simulink model "lqr_period_with_r_and_d_simulink"  (R2015a)
settings: Solver=ode45  SolverMode=SingleTasking  StartTime=0.0  StopTime=simu.time  RelTol=1e-3
values from neighbouring files (symbols this model uses):
  plant = tf([10],[tau 1])    [lqr_period_with_abitary_reference.m]
undefined symbols (not defined in the file or in its folder): simu
undefined symbols (not defined in the file): parameters
libraries: simulink x1
settings Model: CovSFcnEnable=off  ExtModeTrigMode=oneshot  ExtModeArmWhenConnect=off  Creator=The MathWorks Inc.  LastModifiedBy=Xiaotian
settings DataIOCC: LimitDataPoints=off  SaveOutput=off  SignalLogging=off  DSMLogging=off  SaveTime=off  SignalLoggingName=sigsOut
settings OptimizationCC: BooleanDataType=off  ExpressionDepthLimit=2147483647  InitFltsAndDblsToZero=on
settings DebuggingCC: SaveWithParameterizedLinksMsg=none  UnderspecifiedInitializationDetection=Classic  MergeDetectMultiDrivingBlocksExec=none  SignalResolutionControl=TryResolveAllWithWarning  MultiTaskDSMMsg=warning  MultiTaskCondExecSysMsg=none  IntegerOverflowMsg=none  FcnCallInpInsideContextMsg=UseLocalSettings  StateNameClashWarn=warning  IntegerSaturationMsg=none
settings HardwareCC: TargetUnknown=on
settings GRTTargetCC: TargetFcnLib=ansi_tfl_tmw.mat  CombineOutputUpdateFcns=off  GRTInterface=on

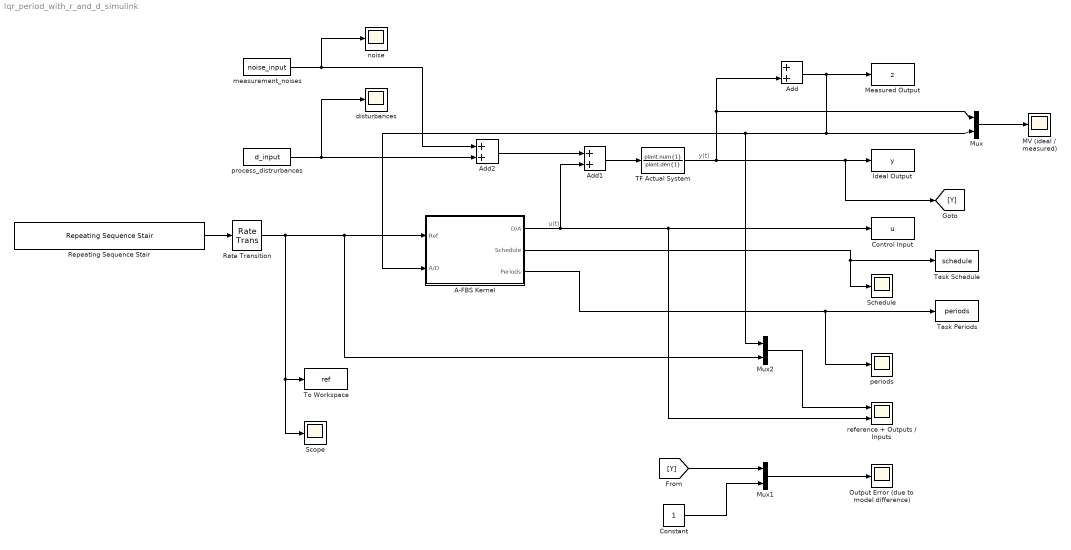
== system lqr_period_with_r_and_d_simulink ==
  note: u(t)
  note: y(t)
  A-FBS Kernel : Subsystem  mask{afbs_para=parameters}
      mask prompts: afbs_para "A-FBS Parameters"
  Add : Sum
  Add1 : Sum
  Add2 : Sum
  Constant : Constant
  Control Input : ToWorkspace  VariableName=u  SampleTime=simu.samlping_time
      settings: MaxDataPoints=Inf
  Ideal Output : ToWorkspace  VariableName=y  SampleTime=simu.samlping_time
      settings: MaxDataPoints=Inf
  MV (ideal / measured) : Scope
      settings: TimeRange=10  YMin=-1.5  YMax=1.75  DataFormat=Structure
  Measured Output : ToWorkspace  VariableName=z  SampleTime=simu.samlping_time
      settings: MaxDataPoints=Inf
  Mux : Mux  Inputs=2
  Mux1 : Mux  Inputs=2
  Mux2 : Mux  Inputs=2
  Output Error (due to model difference) : Scope
      settings: TimeRange=10  YMin=-29.95  YMax=-29.6  SaveName=ScopeData2  DataFormat=Structure  SampleInput=on  SampleTime=simu.samlping_time
  Rate Transition : RateTransition
  Repeating Sequence Stair : simulink/Sources/Repeating Sequence Stair  OutValues=ref_sequence'  tsamp=ref_sampling_time  OutMin=[]  OutMax=[]  OutDataTypeStr=double  OutputDataTypeScalingMode=double  OutDataType=fixdt(0,8)  ConRadixGroup=Best Precision: Vector-wise  OutScaling=2^-12
  Schedule : Scope
      settings: TimeRange=10  YMin=-29.95  YMax=-29.6  SaveName=ScopeData5  DataFormat=Structure  SampleInput=on  SampleTime=simu.samlping_time
  Scope : Scope
      settings: YMin=0.95  YMax=1.05  SaveName=ScopeData7
  TF Actual System : TransferFcn  Numerator=plant.num{1}  Denominator=plant.den{1}
  Task Periods : ToWorkspace  VariableName=periods  SampleTime=simu.samlping_time
      settings: MaxDataPoints=Inf
  Task Schedule : ToWorkspace  VariableName=schedule  SampleTime=simu.samlping_time
      settings: MaxDataPoints=Inf
  To Workspace : ToWorkspace  VariableName=ref  SampleTime=simu.samlping_time
  disturbances : Scope
      settings: TimeRange=10  YMin=-29.95  YMax=-29.6  SaveName=ScopeData4  DataFormat=Structure  SampleInput=on  SampleTime=simu.samlping_time
  measurement_noises : FromWorkspace  VariableName=noise_input  SampleTime=0
  noise : Scope
      settings: TimeRange=10  YMin=-29.95  YMax=-29.6  SaveName=ScopeData3  DataFormat=Structure  SampleInput=on  SampleTime=simu.samlping_time
  periods : Scope
      settings: TimeRange=10  YMin=0.00095  YMax=0.00105  SaveName=ScopeData6  DataFormat=Structure  SampleInput=on  SampleTime=simu.samlping_time
  process_distrurbances : FromWorkspace  VariableName=d_input  SampleTime=0
  reference + Outputs / Inputs : Scope  NumInputPorts=2
      settings: TimeRange=1.022054868208716  YMin=-1~-0.1  YMax=7~0.7000000000000001  DataFormat=Structure  SampleInput=on  SampleTime=simu.samlping_time
  wires:
  A-FBS Kernel/1(D/A) -> reference + Outputs / Inputs/2, Control Input/1, Add1/2
  TF Actual System/1 -> Add/2, Mux/1, [Y], Ideal Output/1
  Repeating Sequence Stair/1 -> Rate Transition/1
  Add/1 -> Mux2/1, A-FBS Kernel/2(A/D), Mux/2, Measured Output/1
  measurement_noises/1 -> Add2/1, noise/1
  Add1/1 -> TF Actual System/1
  process_distrurbances/1 -> disturbances/1, Add2/2
  Mux/1 -> MV (ideal / measured)/1
  Mux1/1 -> Output Error (due to model difference)/1
  [Y] -> Mux1/1
  Mux2/1 -> reference + Outputs / Inputs/1
  A-FBS Kernel/3(Periods) -> Task Periods/1, periods/1
  A-FBS Kernel/2(Schedule) -> Schedule/1, Task Schedule/1
  Rate Transition/1 -> Scope/1, To Workspace/1, Mux2/2, A-FBS Kernel/1(Ref)
  Constant/1 -> Mux1/2
  Add2/1 -> Add1/1

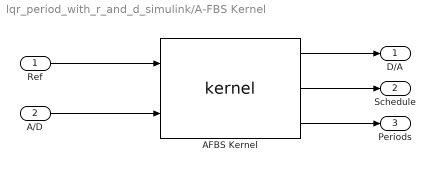
== system lqr_period_with_r_and_d_simulink/A-FBS Kernel ==
  Ref : Inport
  A/D : Inport  Port=2
  AFBS Kernel : S-Function  FunctionName=kernel  Parameters=afbs_para
  D/A : Outport
  Schedule : Outport  Port=2
  Periods : Outport  Port=3
  wires:
  Ref/1 -> AFBS Kernel/1
  A/D/1 -> AFBS Kernel/2
  AFBS Kernel/2 -> Schedule/1
  AFBS Kernel/1 -> D/A/1
  AFBS Kernel/3 -> Periods/1
